simulink model "lab3sim"  (R2020a)
settings: Solver=VariableStepAuto  StartTime=0.0  StopTime=300  RelTol=1e-6
settings Model: Creator=ariana  LastModifiedBy=ariana

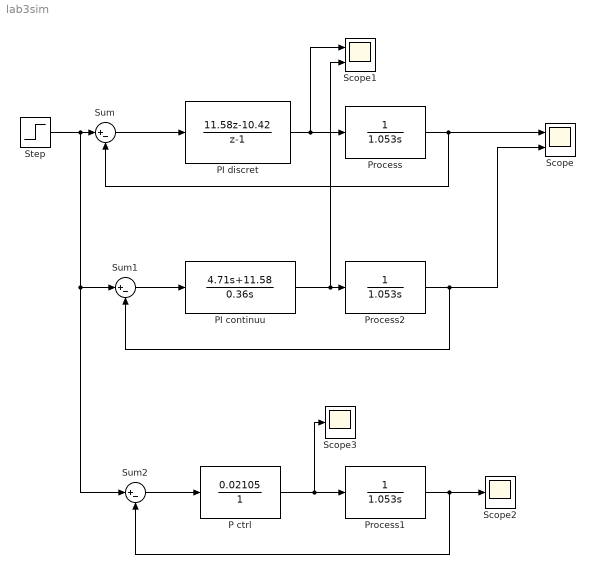
== system lab3sim ==
  P ctrl : TransferFcn  Numerator=[0.02105]  Denominator=[0 1]
  PI continuu : TransferFcn  Numerator=[4.71 11.58]  Denominator=[0.36 0]
  PI discret : DiscreteTransferFcn  Numerator=[11.58 -10.42]  Denominator=[1 -1]  SampleTime=0.036
  Process : TransferFcn  Denominator=[1.053 0]
  Process1 : TransferFcn  Denominator=[1.053 0]
  Process2 : TransferFcn  Denominator=[1.053 0]
  Scope : Scope  NumInputPorts=2
  Scope1 : Scope  NumInputPorts=2
  Scope2 : Scope
  Scope3 : Scope
  Step : Step  Time=0  SampleTime=0
  Sum : Sum  Inputs=|+-
  Sum1 : Sum  Inputs=|+-
  Sum2 : Sum  Inputs=|+-
  wires:
  PI discret/1 -> Scope1/1, Process/1
  Process/1 -> Scope/1, Sum/2
  Sum/1 -> PI discret/1
  Step/1 -> Sum2/1, Sum1/1, Sum/1
  PI continuu/1 -> Scope1/2, Process2/1
  Sum1/1 -> PI continuu/1
  Process2/1 -> Scope/2, Sum1/2
  P ctrl/1 -> Scope3/1, Process1/1
  Sum2/1 -> P ctrl/1
  Process1/1 -> Scope2/1, Sum2/2
